simulink model "NonLinearStabSystem"  (Simulink 8.2)
settings: Solver=ode4  SolverMode=SingleTasking  StartTime=0.0  StopTime=Tend  FixedStep=h  RelTol=1e-3
values from neighbouring files (symbols this model uses):
  dU = 0    [Analysis_of_a_Nonlinear_Electromechanical_Plant.m]
  J = 0.5e-5    (= 5e-06)    [Analysis_of_a_Nonlinear_Electromechanical_Plant.m]
  Ke = 0.05    [Analysis_of_a_Nonlinear_Electromechanical_Plant.m]
  Km = Ke    (= 0.05)    [Analysis_of_a_Nonlinear_Electromechanical_Plant.m]
  Kpc = 3    [Analysis_of_a_Nonlinear_Electromechanical_Plant.m]
  Kvf = 0.00000    (= 0)    [Analysis_of_a_Nonlinear_Electromechanical_Plant.m]
  M_L = 0.0    (= 0)    [Analysis_of_a_Nonlinear_Electromechanical_Plant.m]
  Mdf = 0.000    (= 0)    [Analysis_of_a_Nonlinear_Electromechanical_Plant.m]
  Ra = 10    [Analysis_of_a_Nonlinear_Electromechanical_Plant.m]
  t_L = Tend/2    (= 0.75)    [Analysis_of_a_Nonlinear_Electromechanical_Plant.m]
  Ta = La/Ra    (= 0.01)    [Analysis_of_a_Nonlinear_Electromechanical_Plant.m]
  Tpc = 0.001    [Analysis_of_a_Nonlinear_Electromechanical_Plant.m]
undefined symbols (not defined in the file or in its folder): g, Kcr, Kcs, Kvr, Kvs, Tcr, Tvr, Umax
settings Model: Creator=RIS  LastModifiedBy=RIS
settings DataIOCC: SignalLoggingSaveFormat=Dataset
settings OptimizationCC: ExpressionDepthLimit=128
settings DebuggingCC: FcnCallInpInsideContextMsg=EnableAllAsError  StateNameClashWarn=none
settings GRTTargetCC: CombineOutputUpdateFcns=on  GRTInterface=off

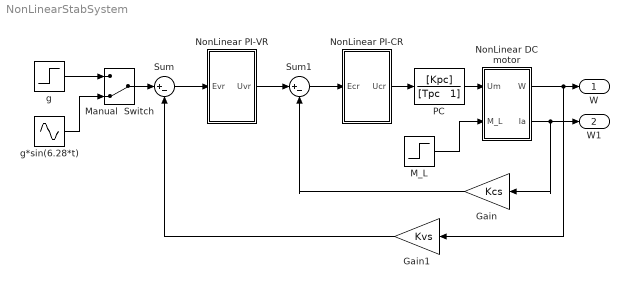
== system NonLinearStabSystem ==
  " NonLinear DC motor" : Subsystem
  " NonLinear PI-CR" : Subsystem
  " NonLinear PI-VR" : Subsystem
  Gain : Gain  Gain=Kcs
  Gain1 : Gain  Gain=Kvs
  M_L : Step  Time=t_L  After=M_L  SampleTime=0
  Manual  Switch : ManualSwitch  CurrentSetting=0
  PC : TransferFcn  Numerator=[Kpc]  Denominator="[Tpc   1]"
  Sum : Sum  Inputs=|+-
  Sum1 : Sum  Inputs=|+-
  g : Step  Time=0  After=g  SampleTime=0
  g*sin(6.28*t) : Sin  Amplitude=g  Frequency=6.28  SampleTime=0
  W : Outport
  W1 : Outport  Port=2
  wires:
  g/1 -> Manual  Switch/1
  g*sin(6.28*t)/1 -> Manual  Switch/2
  PC/1 -> " NonLinear DC motor"/1("Um ")
  M_L/1 -> " NonLinear DC motor"/2(M_L)
  Manual  Switch/1 -> Sum/1
  Sum/1 -> " NonLinear PI-VR"/1("Evr ")
  " NonLinear PI-VR"/1(Uvr) -> Sum1/1
  Sum1/1 -> " NonLinear PI-CR"/1("Ecr ")
  " NonLinear PI-CR"/1(Ucr) -> PC/1
  " NonLinear DC motor"/2(Ia) -> Gain/1, W1/1
  " NonLinear DC motor"/1(W) -> Gain1/1, W/1
  Gain/1 -> Sum1/2
  Gain1/1 -> Sum/2

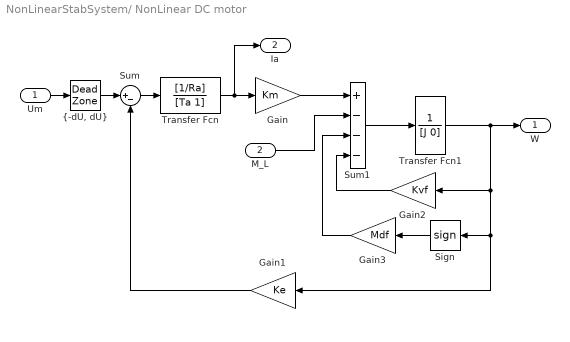
== system NonLinearStabSystem/ NonLinear DC motor ==
  "Um " : Inport
  M_L : Inport  Port=2
  Gain : Gain  Gain=Km
  Gain1 : Gain  Gain=Ke
  Gain2 : Gain  Gain=Kvf
  Gain3 : Gain  Gain=Mdf
  Sign : Signum
  Sum : Sum  Inputs=|+-
  Sum1 : Sum  Inputs=+---
  Transfer Fcn : TransferFcn  Numerator=[1/Ra]  Denominator=[Ta 1]
  Transfer Fcn1 : TransferFcn  Denominator=[J 0]
  "{-dU, dU}" : DeadZone  LowerValue=-dU  UpperValue=dU  SaturateOnIntegerOverflow=on
  W : Outport
  Ia : Outport  Port=2
  wires:
  Sum/1 -> Transfer Fcn/1
  Transfer Fcn/1 -> Gain/1, Ia/1
  Gain/1 -> Sum1/1
  Sum1/1 -> Transfer Fcn1/1
  Gain1/1 -> Sum/2
  M_L/1 -> Sum1/2
  "Um "/1 -> "{-dU, dU}"/1
  "{-dU, dU}"/1 -> Sum/1
  Gain2/1 -> Sum1/4
  Transfer Fcn1/1 -> Gain2/1, Gain1/1, Sign/1, W/1
  Sign/1 -> Gain3/1
  Gain3/1 -> Sum1/3

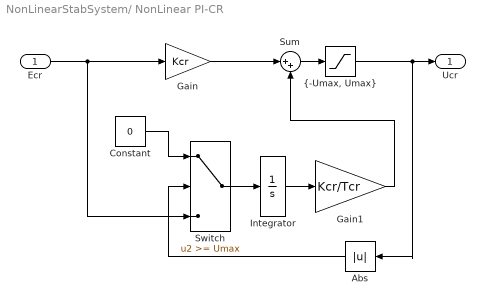
== system NonLinearStabSystem/ NonLinear PI-CR ==
  "Ecr " : Inport
  Abs : Abs
  Constant : Constant  Value=0
  Gain : Gain  Gain=Kcr
  Gain1 : Gain  Gain=Kcr/Tcr
  Integrator : Integrator
  Sum : Sum  Inputs=|++
  Switch : Switch  Threshold=Umax
  "{-Umax, Umax}" : Saturate  UpperLimit=Umax  LowerLimit=-Umax
  Ucr : Outport
  wires:
  "Ecr "/1 -> Switch/3, Gain/1
  Constant/1 -> Switch/1
  Integrator/1 -> Gain1/1
  Switch/1 -> Integrator/1
  Gain/1 -> Sum/1
  Gain1/1 -> Sum/2
  Sum/1 -> "{-Umax, Umax}"/1
  "{-Umax, Umax}"/1 -> Abs/1, Ucr/1
  Abs/1 -> Switch/2

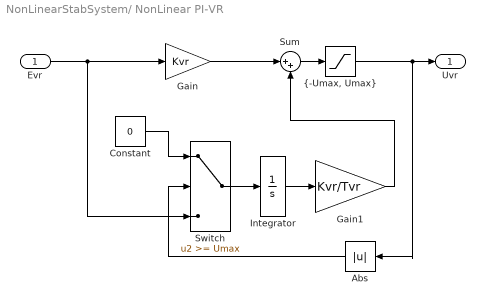
== system NonLinearStabSystem/ NonLinear PI-VR ==
  "Evr " : Inport
  Abs : Abs
  Constant : Constant  Value=0
  Gain : Gain  Gain=Kvr
  Gain1 : Gain  Gain=Kvr/Tvr
  Integrator : Integrator
  Sum : Sum  Inputs=|++
  Switch : Switch  Threshold=Umax
  "{-Umax, Umax}" : Saturate  UpperLimit=Umax  LowerLimit=-Umax
  Uvr : Outport
  wires:
  "Evr "/1 -> Switch/3, Gain/1
  Constant/1 -> Switch/1
  Integrator/1 -> Gain1/1
  Switch/1 -> Integrator/1
  Gain/1 -> Sum/1
  Gain1/1 -> Sum/2
  Sum/1 -> "{-Umax, Umax}"/1
  "{-Umax, Umax}"/1 -> Abs/1, Uvr/1
  Abs/1 -> Switch/2
